simulink model "Linealizacion"  (R2024a)
settings: Solver=VariableStepAuto  StartTime=0.0  StopTime=20.0  MaxStep=0.01  RelTol=1e-3
settings Model: Creator=alfre
settings RTWCC: GPUComputeCapability=3.5

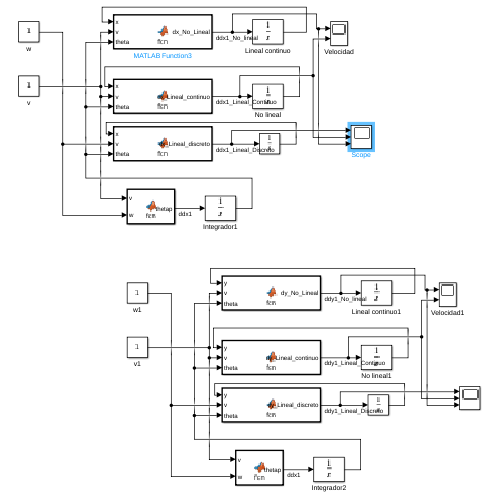
[thumbnail: Simulink's stored preview of the top-level diagram]
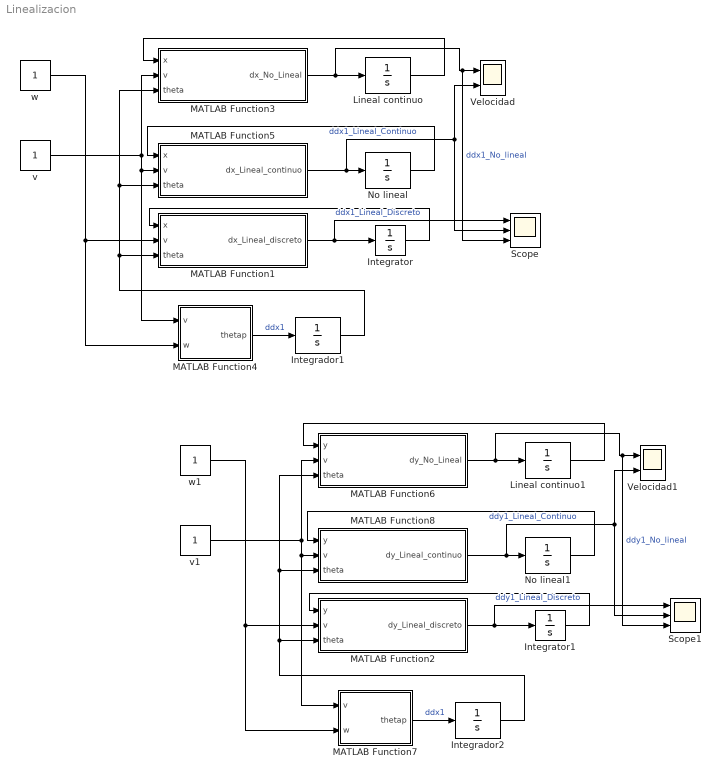
== system Linealizacion ==
  Integrador1 : Integrator  ContinuousStateAttributes="\"dx\""
  Integrador2 : Integrator  ContinuousStateAttributes="\"dx\""
  Integrator : Integrator
  Integrator1 : Integrator
  Lineal continuo : Integrator  ContinuousStateAttributes="\"dx\""
  Lineal continuo1 : Integrator  ContinuousStateAttributes="\"dx\""
  MATLAB Function1 : MATLAB Function  TreatAsAtomicUnit=on
  MATLAB Function2 : MATLAB Function  TreatAsAtomicUnit=on
  MATLAB Function3 : MATLAB Function  TreatAsAtomicUnit=on
  MATLAB Function4 : MATLAB Function  TreatAsAtomicUnit=on
  MATLAB Function5 : MATLAB Function  TreatAsAtomicUnit=on
  MATLAB Function6 : MATLAB Function  TreatAsAtomicUnit=on
  MATLAB Function7 : MATLAB Function  TreatAsAtomicUnit=on
  MATLAB Function8 : MATLAB Function  TreatAsAtomicUnit=on
  No lineal : Integrator  ContinuousStateAttributes="\"dx\""
  No lineal1 : Integrator  ContinuousStateAttributes="\"dx\""
  Scope : Scope  NumInputPorts=3
  Scope1 : Scope  NumInputPorts=3
  Velocidad : Scope  NumInputPorts=2
  Velocidad1 : Scope  NumInputPorts=2
  v : Constant
  v1 : Constant
  w : Constant
  w1 : Constant
  wires:
  Lineal continuo/1 -> MATLAB Function3/1(x)
  Integrador1/1 -> MATLAB Function1/3(theta), MATLAB Function5/3(theta), MATLAB Function3/3(theta)
  MATLAB Function3/1(dx_No_Lineal) -> Scope/3, Velocidad/1, Lineal continuo/1  "ddx1_No_lineal"
  No lineal/1 -> MATLAB Function5/1(x)
  w/1 -> MATLAB Function1/2(v), MATLAB Function4/2(w)
  MATLAB Function5/1(dx_Lineal_continuo) -> Velocidad/2, Scope/2, No lineal/1  "ddx1_Lineal_Continuo"
  MATLAB Function4/1(thetap) -> Integrador1/1  "ddx1"
  v/1 -> MATLAB Function3/2(v), MATLAB Function5/2(v), MATLAB Function4/1(v)
  MATLAB Function1/1(dx_Lineal_discreto) -> Scope/1, Integrator/1  "ddx1_Lineal_Discreto"
  Integrator/1 -> MATLAB Function1/1(x)
  v1/1 -> MATLAB Function6/2(v), MATLAB Function8/2(v), MATLAB Function7/1(v)
  MATLAB Function8/1(dy_Lineal_continuo) -> Velocidad1/2, Scope1/2, No lineal1/1  "ddy1_Lineal_Continuo"
  Integrator1/1 -> MATLAB Function2/1(y)
  w1/1 -> MATLAB Function2/2(v), MATLAB Function7/2(w)
  MATLAB Function2/1(dy_Lineal_discreto) -> Scope1/1, Integrator1/1  "ddy1_Lineal_Discreto"
  MATLAB Function6/1(dy_No_Lineal) -> Scope1/3, Velocidad1/1, Lineal continuo1/1  "ddy1_No_lineal"
  No lineal1/1 -> MATLAB Function8/1(y)
  MATLAB Function7/1(thetap) -> Integrador2/1  "ddx1"
  Integrador2/1 -> MATLAB Function2/3(theta), MATLAB Function8/3(theta), MATLAB Function6/3(theta)
  Lineal continuo1/1 -> MATLAB Function6/1(y)

== matlab function Linealizacion/MATLAB Function1 ==
  data: x input; v input; dx_Lineal_discreto output; theta input
function dx_Lineal_discreto = fcn(x, v, theta)

dx_Lineal_discreto = x -v*sin(theta)*theta;

== matlab function Linealizacion/MATLAB Function2 ==
  data: y input; v input; dy_Lineal_discreto output; theta input
function dy_Lineal_discreto = fcn(y, v, theta)

dy_Lineal_discreto = y+v*cos(theta)*theta

== matlab function Linealizacion/MATLAB Function6 ==
  data: y input; v input; dy_No_Lineal output; theta input
function dy_No_Lineal = fcn(y, v, theta)
dy_No_Lineal= v*sin(theta);

== matlab function Linealizacion/MATLAB Function3 ==
  data: x input; v input; dx_No_Lineal output; theta input
function dx_No_Lineal = fcn(x, v, theta)
dx_No_Lineal= v*cos(theta);

== matlab function Linealizacion/MATLAB Function4 ==
  data: v input; w input; thetap output
function thetap = fcn(v,w)
r=1;
w=v/r;
thetap=w;

== matlab function Linealizacion/MATLAB Function5 ==
  data: x input; v input; dx_Lineal_continuo output; theta input
function dx_Lineal_continuo = fcn(x, v, theta)

dx_Lineal_continuo = -v*sin(theta)*theta;

== matlab function Linealizacion/MATLAB Function7 ==
  data: v input; w input; thetap output
function thetap = fcn(v,w)
r=1;
w=v/r;
thetap=w;

== matlab function Linealizacion/MATLAB Function8 ==
  data: y input; v input; dy_Lineal_continuo output; theta input
function dy_Lineal_continuo = fcn(y, v, theta)
dy_Lineal_continuo = v*cos(theta)*theta
